simulink model "Final_Model_7"  (Simulink 10.1)
settings: Solver=ode3  StartTime=0.0  StopTime=5  FixedStep=10e-6  RelTol=1e-3
undefined symbols (not defined in the file): B, J, K, L, P, R
libraries: powerlib x12, simulink x7
settings Model: Creator=SONY  LastModifiedBy=user
settings DataIOCC: SaveFormat=StructureWithTime  ReturnWorkspaceOutputs=on
settings DebuggingCC: UnderspecifiedInitializationDetection=Simplified  MergeDetectMultiDrivingBlocksExec=error  SFUnexpectedBacktrackingDiag=error  SFNoUnconditionalDefaultTransitionDiag=error
settings HardwareCC: ProdBitPerPointer=64  ProdLargestAtomicFloat=Float  ProdIntDivRoundTo=Zero  ProdEndianess=LittleEndian  ProdHWDeviceType=Specified
settings ModelReferenceCC: PropagateSignalLabelsOutOfModel=on
settings SFSimCC: SimUseLocalCustomCode=on
settings RTWCC: RTWUseLocalCustomCode=on
settings GRTTargetCC: TargetLangStandard=C99 (ISO)  CombineOutputUpdateFcns=on  GRTInterface=off
settings ConfigComp: CovMetricSettings=dwe  CovHtmlReporting=off  CovSaveCumulativeToWorkspaceVar=off  CovSaveSingleToWorkspaceVar=off  CovExternalEMLEnable=on

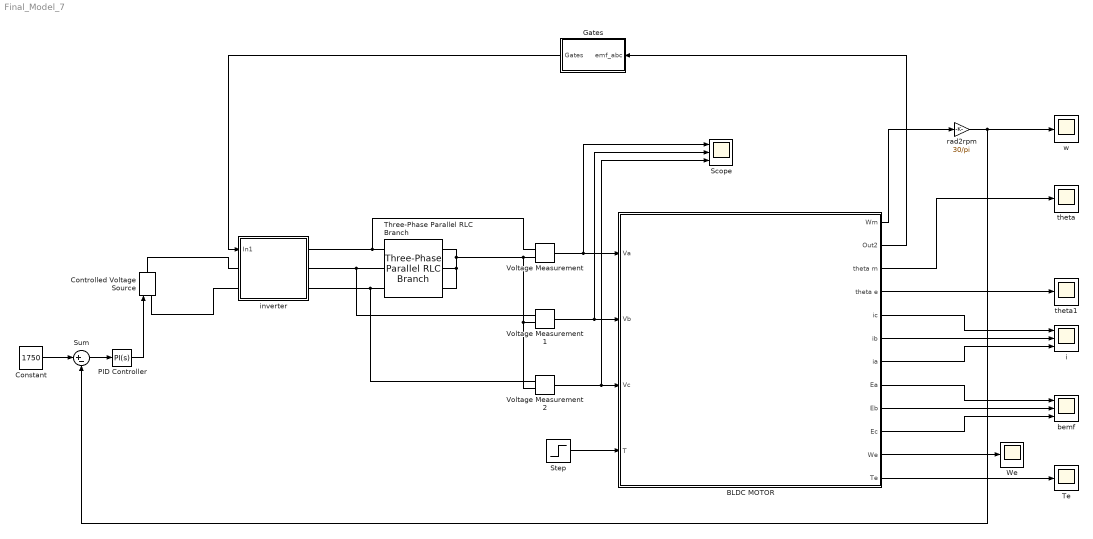
== system Final_Model_7 ==
  BLDC MOTOR : Subsystem
  Constant : Constant  Value=1750
  Controlled Voltage Source : powerlib/Electrical Sources/Controlled Voltage Source  Initialize=on  Source_Type=DC  Amplitude=300  Phase=0  Frequency=50  Measurements=Voltage
  Gates : Subsystem
  PID Controller : simulink/Continuous/PID Controller  Controller=PI  Form=Parallel  TimeDomain=Continuous-time  UseExternalTs=off  SampleTime=-1  IntegratorMethod=Forward Euler  FilterMethod=Forward Euler  ControllerParametersSource=internal  P=0.000000001  I=33.4987439489544  D=0  UseFilter=on  N=100  TunerSelectOption=Frequency Response Based  InitialConditionSource=internal  InitialConditionForIntegrator=0  InitialConditionForFilter=0  DifferentiatorICPrevScaledInput=0  ExternalReset=none  TrackingMode=off  Kt=1  LimitOutput=off  UpperSaturationLimit=inf  LowerSaturationLimit=-inf  LinearizeAsGain=on  AntiWindupMode=none  Kb=1  POutMin=[]  POutMax=[]  IOutMin=[]  IOutMax=[]  DOutMin=[]  DOutMax=[]  NOutMin=[]  NOutMax=[]  SumOutMin=[]  SumOutMax=[]  SaturationOutMin=[]  SaturationOutMax=[]  PParamMin=[]  PParamMax=[]  IParamMin=[]  IParamMax=[]  DParamMin=[]  DParamMax=[]  NParamMin=[]  NParamMax=[]  KbParamMin=[]  KbParamMax=[]  KtParamMin=[]  KtParamMax=[]  KbOutMin=[]  KbOutMax=[]  KtOutMin=[]  KtOutMax=[]  IntegratorOutMin=[]  IntegratorOutMax=[]  FilterOutMin=[]  FilterOutMax=[]  SumI1OutMin=[]  SumI1OutMax=[]  SumI2OutMin=[]  SumI2OutMax=[]  SumI3OutMin=[]  SumI3OutMax=[]  SumI4OutMin=[]  SumI4OutMax=[]  SumDOutMin=[]  SumDOutMax=[]  DifferentiatorOutMin=[]  DifferentiatorOutMax=[]  FilterDiffOutCoefMin=[]  FilterDiffOutCoefMax=[]  ReciprocalOutMin=[]  ReciprocalOutMax=[]  SumDenOutMin=[]  SumDenOutMax=[]  SumNumOutMin=[]  SumNumOutMax=[]  DivideOutMin=[]  DivideOutMax=[]  UdiffTsProdOutMin=[]  UdiffTsProdOutMax=[]  NTsProdOutMin=[]  NTsProdOutMax=[]  UintegralTsProdOutMin=[]  UintegralTsProdOutMax=[]  UngainTsProdOutMin=[]  UngainTsProdOutMax=[]  IntegratorContinuousStateAttributes=''  IntegratorStateMustResolveToSignalObject=off  IntegratorRTWStateStorageClass=Auto  FilterContinuousStateAttributes=''  FilterStateMustResolveToSignalObject=off  FilterRTWStateStorageClass=Auto  ParallelPVariant=InternalParameters  IdealPVariant=Disabled  IVariant=InternalParameters  DVariant=Disabled  IntegratorVariant=Continuous  SatVariant=Disabled  AWVariant=Passthrough  PCopyVariant=Disabled  TRVariant=Disabled  FdbkBlocksVariant=Forward  IdealPFdbkVariant=Disabled  SatFdbkVariant=Disabled  DerivativeFilterVariant=Disabled  NVariant=Disabled  NCopyVariant=Disabled_SignalSpec  FilterICVariant=Disabled  IntegratorICVariant=InternalICs  ExternalResetVariant=Disabled  TRSumVariant=Passthrough  SumFdbkVariant=Disabled  SumVariant=Sum_PI  TsampFilterVariant=InternalTs  TsampNgainVariant=Passthrough  TsampIntegralVariant=Passthrough
  Scope : Scope  NumInputPorts=3
  Step : Step  Time=2  After=3  SampleTime=0
  Sum : Sum  Inputs=|+-
  Te : Scope
  Three-Phase Parallel RLC Branch : powerlib/Elements/Three-Phase Parallel RLC Branch  LConnTagsString=A|B|C  RConnTagsString=A|B|C  BranchType=R  Resistance=1  Inductance=1e-3  Capacitance=1e-6  Measurements=None
      settings: SourceProductBaseCode=PS
  Voltage Measurement : powerlib/Measurements/Voltage Measurement  PhasorSimulation=off  OutputType=Complex  PSBequivalent=0
  Voltage Measurement1 : powerlib/Measurements/Voltage Measurement  PhasorSimulation=off  OutputType=Complex  PSBequivalent=0
  Voltage Measurement2 : powerlib/Measurements/Voltage Measurement  PhasorSimulation=off  OutputType=Complex  PSBequivalent=0
  We : Scope
  bemf : Scope  NumInputPorts=3
  i : Scope  NumInputPorts=3
  inverter : Subsystem
  rad2rpm : Gain  Gain=30/pi
  theta : Scope
  theta1 : Scope
  w : Scope
  wires:
  Voltage Measurement/1 -> BLDC MOTOR/1(Va), Scope/1
  Voltage Measurement1/1 -> Scope/2, BLDC MOTOR/2(Vb)
  Voltage Measurement2/1 -> Scope/3, BLDC MOTOR/3(Vc)
  Step/1 -> BLDC MOTOR/4(T)
  BLDC MOTOR/1(Wm) -> rad2rpm/1
  BLDC MOTOR/2(Out2) -> Gates/1("emf_abc ")
  BLDC MOTOR/3(theta m) -> theta/1
  BLDC MOTOR/4(theta e) -> theta1/1
  BLDC MOTOR/5(ic) -> i/1
  BLDC MOTOR/6(ib) -> i/2
  BLDC MOTOR/7(ia) -> i/3
  BLDC MOTOR/8(Ea) -> bemf/1
  BLDC MOTOR/9(Eb) -> bemf/2
  BLDC MOTOR/10(Ec) -> bemf/3
  BLDC MOTOR/12(Te) -> Te/1
  Gates/1(Gates) -> inverter/1(In1)
  Constant/1 -> Sum/1
  PID Controller/1 -> Controlled Voltage Source/1
  Sum/1 -> PID Controller/1
  BLDC MOTOR/11(We) -> We/1
  rad2rpm/1 -> w/1, Sum/2
  connections:
  Voltage Measurement2/LConn2 -- Three-Phase Parallel RLC Branch/RConn1 -- Three-Phase Parallel RLC Branch/RConn3 -- Three-Phase Parallel RLC Branch/RConn2 -- Voltage Measurement/LConn2 -- Voltage Measurement1/LConn2
  inverter/RConn1 -- Three-Phase Parallel RLC Branch/LConn1 -- Voltage Measurement/LConn1
  inverter/RConn2 -- Voltage Measurement1/LConn1 -- Three-Phase Parallel RLC Branch/LConn2
  inverter/RConn3 -- Voltage Measurement2/LConn1 -- Three-Phase Parallel RLC Branch/LConn3
  Controlled Voltage Source/RConn1 -- inverter/LConn1
  Controlled Voltage Source/LConn1 -- inverter/LConn2

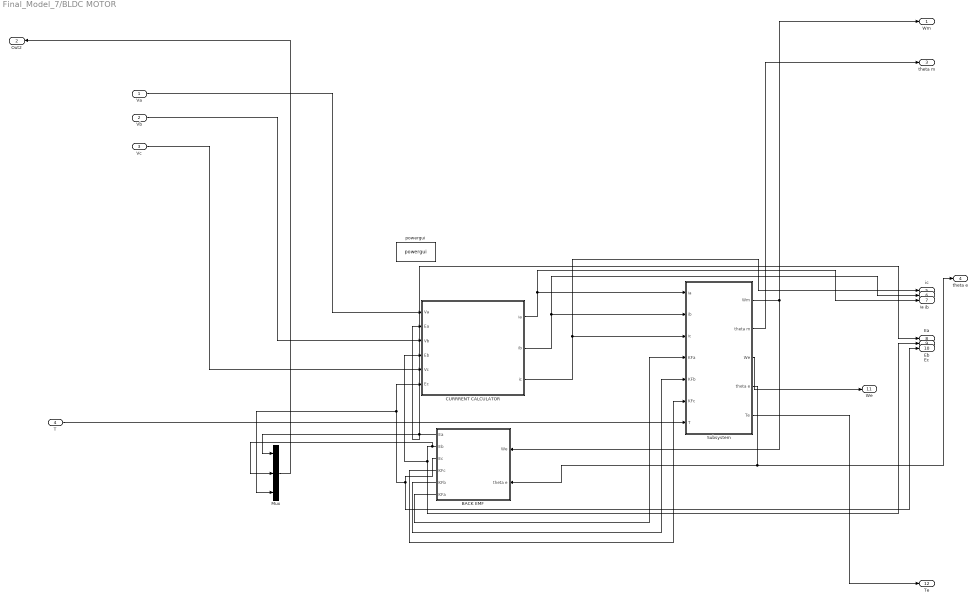
== system Final_Model_7/BLDC MOTOR ==
  Va : Inport
  Vb : Inport  Port=2
  Vc : Inport  Port=3
  T : Inport  Port=4
  BACK EMF : Subsystem
  CURRRENT CALCULATOR : Subsystem
  Mux : Mux  Inputs=3
  Subsystem : Subsystem
  powergui : powerlib/powergui  Priority=1  SimulationMode=Continuous  SampleTime=50e-6  frequency=60  Iterations=50  frequencyindice=0  Pbase=100e6  ErrMax=1e-4  UnitsV=kV  UnitsW=MW  buscounter=0  FunctionMessages=off  echomessages=off  EnableUseOfTLC=off  CurrentSourceSwitches=off  DisableSnubberDevices=off  DisableRonSwitches=off  DisableVfSwitches=off  DisplayEquations=off  AutomaticDiscreteSolvers=off  SolverType=Tustin/Backward Euler (TBE)  Interpol=off  ExternalGateDelay=off  methode=off  Ts=100  x0status=blocks  SPID=on  SwTol=0  HookPort=off  NonlinearTolerance=1e-4  nMaxIteration=100  ContinueOnMaxIteration=off  RestoreLinks=warning  ResistiveCurrentMeasurement=off  Frange=[0:2:500]  Ylog=off  Xlog=on  ShowGrid=off  save=off  variable=ZData  structure=0  ZoomFFT=off  StartTime=0.0  cycles=1  DisplayStyle=1  fundamental=60  FreqAxis=off  MaxFrequency=1000  frequencyindicesteady=1  RmsSteady=1  display=off
  Wm : Outport
  Out2 : Outport  Port=2
  theta m : Outport  Port=3
  theta e : Outport  Port=4
  ic : Outport  Port=5
  ib : Outport  Port=6
  ia : Outport  Port=7
  Ea : Outport  Port=8
  Eb : Outport  Port=9
  Ec : Outport  Port=10
  We : Outport  Port=11
  Te : Outport  Port=12
  wires:
  BACK EMF/5(KFb) -> Subsystem/5(KFb)
  BACK EMF/4(KFc) -> Subsystem/6(KFc)
  Vc/1 -> CURRRENT CALCULATOR/5(Vc)
  Subsystem/4(theta e) -> BACK EMF/2(theta e), theta e/1
  BACK EMF/6(KFa) -> Subsystem/4(KFa)
  BACK EMF/2(Eb) -> Mux/2, Eb/1, CURRRENT CALCULATOR/4(Eb)
  BACK EMF/3(Ec) -> Ec/1, Mux/3, CURRRENT CALCULATOR/6(Ec)
  Subsystem/1(Wm) -> Wm/1, BACK EMF/1(We)
  CURRRENT CALCULATOR/1(ia) -> ia/1, Subsystem/1(ia)
  BACK EMF/1(Ea) -> CURRRENT CALCULATOR/2(Ea), Ea/1, Mux/1
  Vb/1 -> CURRRENT CALCULATOR/3(Vb)
  CURRRENT CALCULATOR/3(ic) -> ic/1, Subsystem/3(ic)
  T/1 -> Subsystem/7(T)
  CURRRENT CALCULATOR/2(ib) -> ib/1, Subsystem/2(ib)
  Subsystem/3(We) -> We/1
  Va/1 -> CURRRENT CALCULATOR/1(Va)
  Mux/1 -> Out2/1
  Subsystem/2(theta m) -> theta m/1
  Subsystem/5(Te) -> Te/1

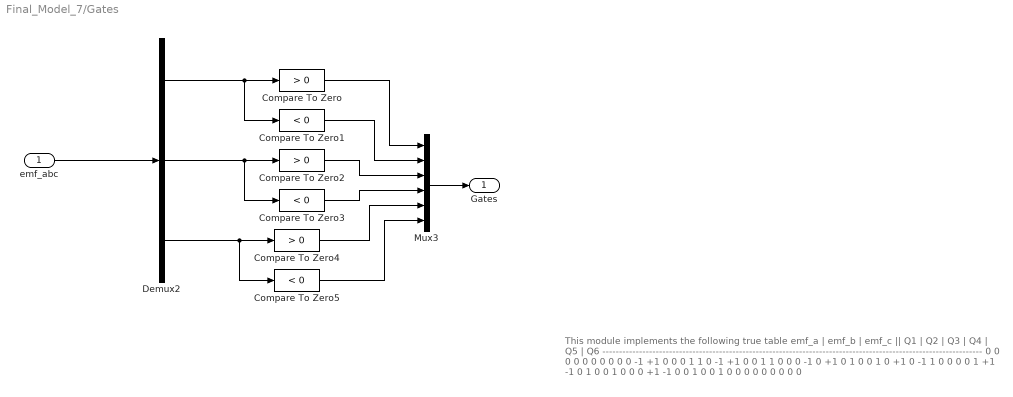
== system Final_Model_7/Gates ==
  note: This module implements the following true table
      |
      |    emf_a   |   emf_b   |   emf_c   ||   Q1   |   Q2   |   Q3   |   Q4   |   Q5   |   Q6
      |     ------------------------------------------------------------------------------------------------------------------
      |       0              0                0            0          0          0           0        0        0
      |       0               -1              +1          0          0          0           1        1        0
      |     -1              +1                0          0          1          1           0        0        0
      |     -1               0               +1          0          1         0           0        1        0
      |    +1               0                -1          1          0          0           0        0        1
      |    +1              -1                0           1          0          0           1        0        0
      |      0              +1               -1           0          0          1           0        0        1
      |     0              0                0             0          0          0           0        0        0
  "emf_abc " : Inport
  Compare To Zero : simulink/Logic and Bit Operations/Compare To Zero  relop=>  OutDataTypeStr=boolean  ZeroCross=off
  Compare To Zero1 : simulink/Logic and Bit Operations/Compare To Zero  relop=<  OutDataTypeStr=boolean  ZeroCross=off
  Compare To Zero2 : simulink/Logic and Bit Operations/Compare To Zero  relop=>  OutDataTypeStr=boolean  ZeroCross=off
  Compare To Zero3 : simulink/Logic and Bit Operations/Compare To Zero  relop=<  OutDataTypeStr=boolean  ZeroCross=off
  Compare To Zero4 : simulink/Logic and Bit Operations/Compare To Zero  relop=>  OutDataTypeStr=boolean  ZeroCross=off
  Compare To Zero5 : simulink/Logic and Bit Operations/Compare To Zero  relop=<  OutDataTypeStr=boolean  ZeroCross=off
  Demux2 : Demux  Outputs=3
  Mux3 : Mux  Inputs=6
  Gates : Outport
  wires:
  "emf_abc "/1 -> Demux2/1
  Mux3/1 -> Gates/1
  Demux2/1 -> Compare To Zero/1, Compare To Zero1/1
  Demux2/2 -> Compare To Zero2/1, Compare To Zero3/1
  Demux2/3 -> Compare To Zero4/1, Compare To Zero5/1
  Compare To Zero/1 -> Mux3/1
  Compare To Zero1/1 -> Mux3/2
  Compare To Zero2/1 -> Mux3/3
  Compare To Zero3/1 -> Mux3/4
  Compare To Zero4/1 -> Mux3/5
  Compare To Zero5/1 -> Mux3/6

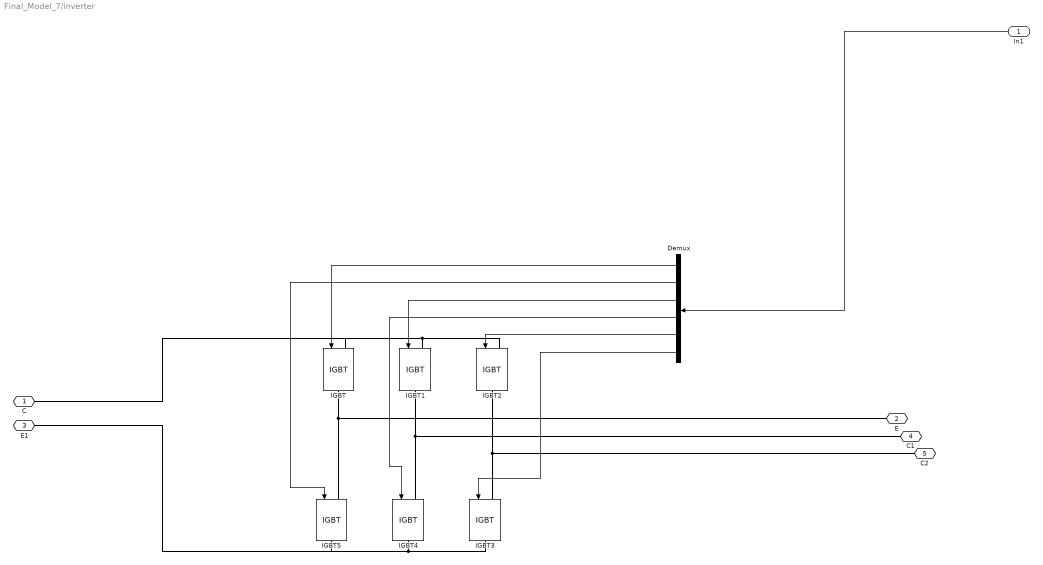
== system Final_Model_7/inverter ==
  In1 : Inport
  Demux : Demux  Outputs=6
  IGBT{,1..5} (6 alike) : powerlib/Power Electronics/IGBT  Ron=0.001  Lon=0  Vf=0  Tf=1e-6  Tt=2e-6  IC=0  Rs=1e5  Cs=inf  Measurements=off
  C : PMIOPort  Side=Left
  E : PMIOPort  Port=2  Side=Right
  E1 : PMIOPort  Port=3  Side=Left
  C1 : PMIOPort  Port=4  Side=Right
  C2 : PMIOPort  Port=5  Side=Right
  wires:
  Demux/1 -> IGBT/1
  Demux/3 -> IGBT1/1
  Demux/4 -> IGBT4/1
  Demux/6 -> IGBT3/1
  Demux/2 -> IGBT5/1
  Demux/5 -> IGBT2/1
  In1/1 -> Demux/1
  connections:
  IGBT5/LConn1 -- E/RConn1 -- IGBT/RConn1
  IGBT1/LConn1 -- C/RConn1 -- IGBT/LConn1 -- IGBT2/LConn1
  IGBT2/RConn1 -- C2/RConn1 -- IGBT3/LConn1
  IGBT4/RConn1 -- E1/RConn1 -- IGBT5/RConn1 -- IGBT3/RConn1
  IGBT1/RConn1 -- C1/RConn1 -- IGBT4/LConn1

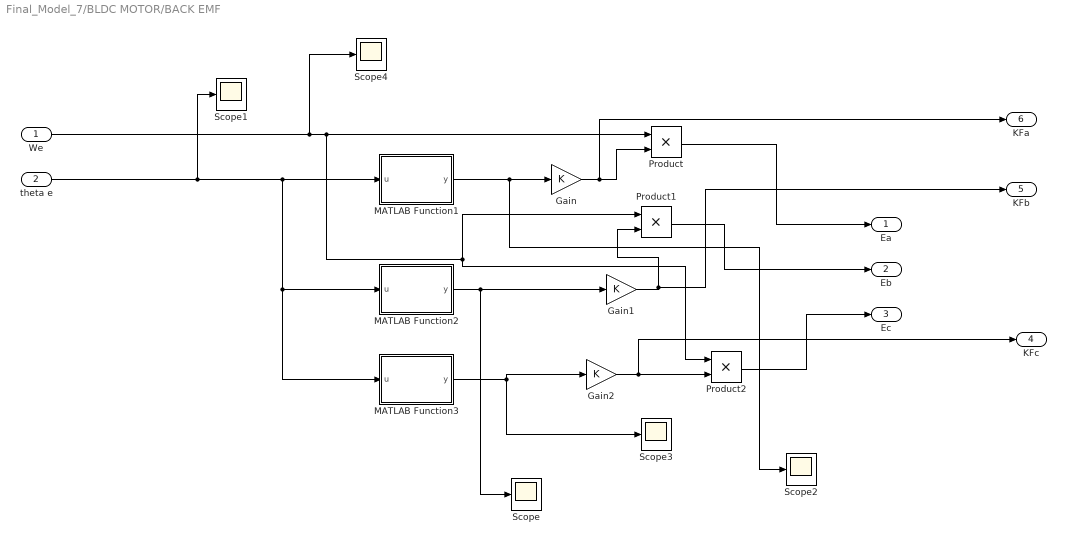
== system Final_Model_7/BLDC MOTOR/BACK EMF ==
  We : Inport
  theta e : Inport  Port=2
  Gain : Gain  Gain=K
  Gain1 : Gain  Gain=K
  Gain2 : Gain  Gain=K
  MATLAB Function1 : MATLAB Function  TreatAsAtomicUnit=on
  MATLAB Function2 : MATLAB Function  TreatAsAtomicUnit=on
  MATLAB Function3 : MATLAB Function  TreatAsAtomicUnit=on
  Product : Product
  Product1 : Product
  Product2 : Product
  Scope{,1..4} (5 alike) : Scope
  Ea : Outport
  Eb : Outport  Port=2
  Ec : Outport  Port=3
  KFc : Outport  Port=4
  KFb : Outport  Port=5
  KFa : Outport  Port=6
  wires:
  We/1 -> Scope4/1, Product1/1, Product2/1, Product/1
  Gain1/1 -> KFb/1, Product1/2
  MATLAB Function3/1(y) -> Scope3/1, Gain2/1
  Gain2/1 -> KFc/1, Product2/2
  MATLAB Function1/1(y) -> Scope2/1, Gain/1
  Gain/1 -> KFa/1, Product/2
  Product/1 -> Ea/1
  MATLAB Function2/1(y) -> Scope/1, Gain1/1
  Product1/1 -> Eb/1
  Product2/1 -> Ec/1
  theta e/1 -> MATLAB Function2/1(u), MATLAB Function3/1(u), MATLAB Function1/1(u), Scope1/1

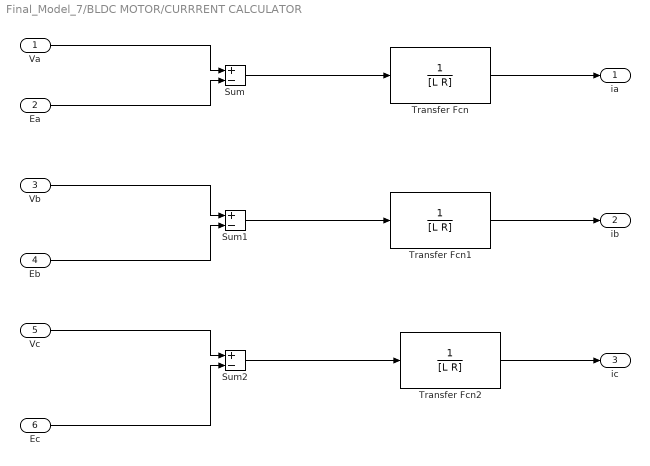
== system Final_Model_7/BLDC MOTOR/CURRRENT CALCULATOR ==
  Va : Inport
  Ea : Inport  Port=2
  Vb : Inport  Port=3
  Eb : Inport  Port=4
  Vc : Inport  Port=5
  Ec : Inport  Port=6
  Sum : Sum  Inputs=+-
  Sum1 : Sum  Inputs=+-
  Sum2 : Sum  Inputs=+-
  Transfer Fcn : TransferFcn  Denominator=[L R]
  Transfer Fcn1 : TransferFcn  Denominator=[L R]
  Transfer Fcn2 : TransferFcn  Denominator=[L R]
  ia : Outport
  ib : Outport  Port=2
  ic : Outport  Port=3
  wires:
  Eb/1 -> Sum1/2
  Vc/1 -> Sum2/1
  Sum/1 -> Transfer Fcn/1
  Sum2/1 -> Transfer Fcn2/1
  Sum1/1 -> Transfer Fcn1/1
  Vb/1 -> Sum1/1
  Ea/1 -> Sum/2
  Va/1 -> Sum/1
  Ec/1 -> Sum2/2
  Transfer Fcn/1 -> ia/1
  Transfer Fcn1/1 -> ib/1
  Transfer Fcn2/1 -> ic/1

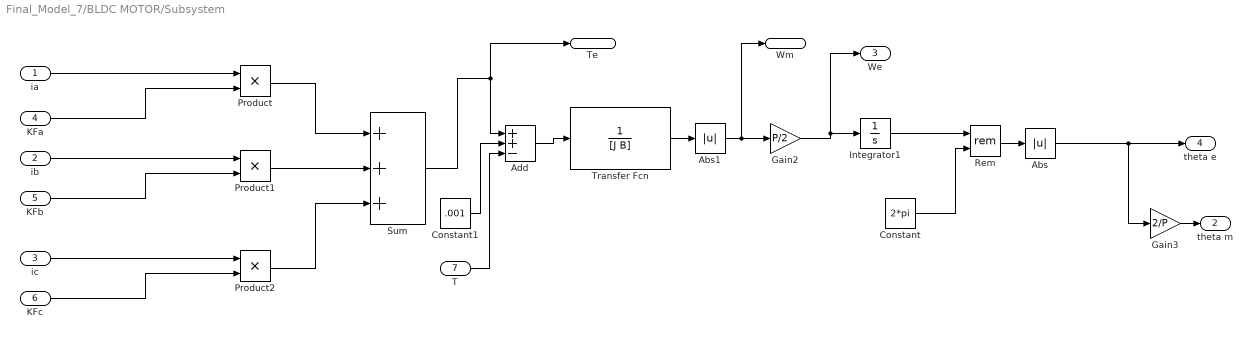
== system Final_Model_7/BLDC MOTOR/Subsystem ==
  ia : Inport
  ib : Inport  Port=2
  ic : Inport  Port=3
  KFa : Inport  Port=4
  KFb : Inport  Port=5
  KFc : Inport  Port=6
  T : Inport  Port=7
  Abs : Abs
  Abs1 : Abs
  Add : Sum  Inputs=++-
  Constant : Constant  Value=2*pi
  Constant1 : Constant  Value=.001
  Gain2 : Gain  Gain=P/2
  Gain3 : Gain  Gain=2/P
  Integrator1 : Integrator
  Product : Product
  Product1 : Product
  Product2 : Product
  Rem : Math  Operator=rem  SignedPower=on  SaturateOnIntegerOverflow=on
  Sum : Sum  Inputs=+++
  Transfer Fcn : TransferFcn  Denominator=[J B]
  Wm : Outport
  theta m : Outport  Port=2
  We : Outport  Port=3
  theta e : Outport  Port=4
  Te : Outport  Port=5
  wires:
  ia/1 -> Product/1
  ib/1 -> Product1/1
  ic/1 -> Product2/1
  KFb/1 -> Product1/2
  KFc/1 -> Product2/2
  Product/1 -> Sum/1
  Product1/1 -> Sum/2
  Product2/1 -> Sum/3
  KFa/1 -> Product/2
  Add/1 -> Transfer Fcn/1
  Gain2/1 -> Integrator1/1, We/1
  Gain3/1 -> theta m/1
  Constant/1 -> Rem/2
  Transfer Fcn/1 -> Abs1/1
  Sum/1 -> Add/1, Te/1
  Integrator1/1 -> Rem/1
  Rem/1 -> Abs/1
  Abs/1 -> Gain3/1, theta e/1
  T/1 -> Add/3
  Abs1/1 -> Gain2/1, Wm/1
  Constant1/1 -> Add/2

== matlab function BLDC MOTOR/BACK EMF/MATLAB Function1 ==
  data: u input double; y output double
function y = fcn(u)
%%codegen

if (0 <= u )&&(u < (pi)/6)
    u = 6*u/pi;
elseif ((pi)/6 <= u )&&(u < 5*pi/6)
    u = 1;
elseif (5*pi/6 <= u )&&(u < (7*pi)/6)
    u = -(6*u/pi)+6;
elseif ((7*pi)/6 <= u)&&(u  < 11*pi/6)
    u = -1;
elseif (11*pi/6 <= u )&&(u < 2*pi)
    u=(6*u/pi)-12;
end

y = u;

== matlab function BLDC MOTOR/BACK EMF/MATLAB Function2 ==
  data: u input double; y output double
function y = fcn(u)
%%codegen

if (0 <= u )&&(u < (pi)/2)
    u = -1;
elseif ((pi)/2 <= u)&&(u  < 5*pi/6)
    u = (6*u/pi)-4;
elseif (5*pi/6 <= u )&&(u < (9*pi)/6)
    u = 1;
elseif ((9*pi)/6 <= u )&&(u < 11*pi/6)
    u = -(6*u/pi)+10;
elseif (11*pi/6 <= u )&&(u < 2*pi)
    u= -1;
end

y = u;

== matlab function BLDC MOTOR/BACK EMF/MATLAB Function3 ==
  data: u input double; y output double
function y = fcn(u)
%%codegen

if (0 <= u )&&(u < (pi)/6)
    u = 1;
elseif ((pi)/6 <= u )&&(u < pi/2)
    u = -(6*u/pi)+2;
elseif (pi/2 <= u )&&(u < (7*pi)/6)
    u = -1;
elseif ((7*pi)/6 <= u )&&(u < 9*pi/6)
    u = (6*u/pi)-8;
elseif (9*pi/6 <= u )&&(u < 2*pi)
    u= 1;
end

y = u;
